simulink model "foc_current_loop_test"  (R2015a)
settings: Solver=ode45  StartTime=0.0  StopTime=0.01  RelTol=1e-3
libraries: simulink x2
settings Model: Creator=user  LastModifiedBy=user

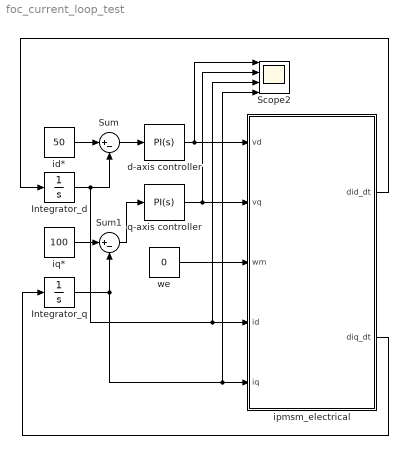
== system foc_current_loop_test ==
  Integrator_d : Integrator
  Integrator_q : Integrator
  Scope2 : Scope  NumInputPorts=4
      settings: YMin=-5~-5~-5~-5  YMax=5~5~5~5  SaveName=ScopeData2
  Sum : Sum  Inputs=|+-
  Sum1 : Sum  Inputs=|+-
  d-axis controller : simulink/Continuous/PID Controller  Controller=PI  TimeDomain=Continuous-time  SampleTime=-1  IntegratorMethod=Forward Euler  FilterMethod=Forward Euler  Form=Parallel  UseFilter=on  ControllerParametersSource=internal  P=0.2827  I=16.6504  D=0  N=100  InitialConditionSource=internal  InitialConditionForIntegrator=0  InitialConditionForFilter=0  ExternalReset=none  LimitOutput=off  UpperSaturationLimit=inf  LowerSaturationLimit=-inf  LinearizeAsGain=on  AntiWindupMode=none  Kb=1  TrackingMode=off  Kt=1  PParamMin=[]  PParamMax=[]  IParamMin=[]  IParamMax=[]  DParamMin=[]  DParamMax=[]  NParamMin=[]  NParamMax=[]  KbParamMin=[]  KbParamMax=[]  KtParamMin=[]  KtParamMax=[]  POutMin=[]  POutMax=[]  IOutMin=[]  IOutMax=[]  DOutMin=[]  DOutMax=[]  NOutMin=[]  NOutMax=[]  KbOutMin=[]  KbOutMax=[]  KtOutMin=[]  KtOutMax=[]  IntegratorOutMin=[]  IntegratorOutMax=[]  FilterOutMin=[]  FilterOutMax=[]  SumOutMin=[]  SumOutMax=[]  SumI1OutMin=[]  SumI1OutMax=[]  SumI2OutMin=[]  SumI2OutMax=[]  SumI3OutMin=[]  SumI3OutMax=[]  SumDOutMin=[]  SumDOutMax=[]  SaturationOutMin=[]  SaturationOutMax=[]  IntegratorContinuousStateAttributes=''  IntegratorStateMustResolveToSignalObject=off  IntegratorRTWStateStorageClass=Auto  FilterContinuousStateAttributes=''  FilterStateMustResolveToSignalObject=off  FilterRTWStateStorageClass=Auto  DifferentiatorICPrevScaledInput=0  DifferentiatorOutMin=[]  DifferentiatorOutMax=[]
  id* : Constant  Value=50
  ipmsm_electrical : MATLAB Function  TreatAsAtomicUnit=on
  iq* : Constant  Value=100
  q-axis controller : simulink/Continuous/PID Controller  Controller=PI  TimeDomain=Continuous-time  SampleTime=-1  IntegratorMethod=Forward Euler  FilterMethod=Forward Euler  Form=Parallel  UseFilter=on  ControllerParametersSource=internal  P=0.8011  I=16.6504  D=0  N=100  InitialConditionSource=internal  InitialConditionForIntegrator=0  InitialConditionForFilter=0  ExternalReset=none  LimitOutput=off  UpperSaturationLimit=inf  LowerSaturationLimit=-inf  LinearizeAsGain=on  AntiWindupMode=none  Kb=1  TrackingMode=off  Kt=1  PParamMin=[]  PParamMax=[]  IParamMin=[]  IParamMax=[]  DParamMin=[]  DParamMax=[]  NParamMin=[]  NParamMax=[]  KbParamMin=[]  KbParamMax=[]  KtParamMin=[]  KtParamMax=[]  POutMin=[]  POutMax=[]  IOutMin=[]  IOutMax=[]  DOutMin=[]  DOutMax=[]  NOutMin=[]  NOutMax=[]  KbOutMin=[]  KbOutMax=[]  KtOutMin=[]  KtOutMax=[]  IntegratorOutMin=[]  IntegratorOutMax=[]  FilterOutMin=[]  FilterOutMax=[]  SumOutMin=[]  SumOutMax=[]  SumI1OutMin=[]  SumI1OutMax=[]  SumI2OutMin=[]  SumI2OutMax=[]  SumI3OutMin=[]  SumI3OutMax=[]  SumDOutMin=[]  SumDOutMax=[]  SaturationOutMin=[]  SaturationOutMax=[]  IntegratorContinuousStateAttributes=''  IntegratorStateMustResolveToSignalObject=off  IntegratorRTWStateStorageClass=Auto  FilterContinuousStateAttributes=''  FilterStateMustResolveToSignalObject=off  FilterRTWStateStorageClass=Auto  DifferentiatorICPrevScaledInput=0  DifferentiatorOutMin=[]  DifferentiatorOutMax=[]
  we : Constant  Value=0
  wires:
  id*/1 -> Sum/1
  Sum/1 -> d-axis controller/1
  d-axis controller/1 -> ipmsm_electrical/1(vd), Scope2/1
  iq*/1 -> Sum1/1
  Integrator_q/1 -> Scope2/4, ipmsm_electrical/5(iq), Sum1/2
  Sum1/1 -> q-axis controller/1
  q-axis controller/1 -> ipmsm_electrical/2(vq), Scope2/2
  we/1 -> ipmsm_electrical/3(wm)
  ipmsm_electrical/2(diq_dt) -> Integrator_q/1
  ipmsm_electrical/1(did_dt) -> Integrator_d/1
  Integrator_d/1 -> Scope2/3, ipmsm_electrical/4(id), Sum/2

== matlab function foc_current_loop_test/ipmsm_electrical ==
  data: vd input; did_dt output; vq input; wm input; id input; iq input; diq_dt output
function [did_dt, diq_dt] = ipmsm_electrical(vd, vq, wm, id, iq)
% BMW i3 IPMSM dq-axis electrical dynamics
% Units: V, rad/s, A, A/s

Rs       = 5.3e-3;    % Stator resistance, Ohm
Ld       = 0.090e-3;  % d-axis inductance, H
Lq       = 0.255e-3;  % q-axis inductance, H
lambda_m = 0.0385;    % PM flux linkage, Wb
p        = 6;         % Pole pairs

we = p*wm;             % electrical angular velocity, rad/s

did_dt = (vd - Rs*id + we*Lq*iq) / Ld;
diq_dt = (vq - Rs*iq - we*(Ld*id + lambda_m)) / Lq;

end
